simulink model "simulink_MPC2"  (R2022b)
settings: Solver=VariableStepAuto  StartTime=0.0  StopTime=Tsim  RelTol=1e-3
values from neighbouring files (symbols this model uses):
  A = [-a_til(2:end)' [eye(length(a_til)-2); zeros(1,length(a_til)-2)]]    [MPC_deadtime.m]    (also in MPC_diofant.m = [1 -0.8]; SS_MPC_irrestrito.m = A'; SS_MPC_restrito.m = A')
  B = [b(2:end)']    [MPC_deadtime.m]    (also in MPC_diofant.m = [0.4 0.6]; SS_MPC_irrestrito.m = B'; SS_MPC_restrito.m = B')
  D = [c(2:end)'-a_til(2:end)']    [MPC_deadtime.m]    (also in SS_MPC_irrestrito.m = D'; SS_MPC_restrito.m = D')
  DistAmplitude = -0.1    [MPC_SS.m]    (also in MPC_ex1_c1.m = 1; MPC_ex1_c2.m = 1; MPC_ex1_c3.m; MPC_ex2_c1.m = -1)
  F = zeros(N,length(a_)-1)    [MPC_SS.m]    (also in MPC_diofant.m = [F; r(2:end)]; MPC_ex1_c1.m; MPC_ex1_c2.m; MPC_ex1_c3.m)
  H = [1 zeros(1,Max-1)]    [MPC_deadtime.m]    (also in SS_MPC_irrestrito.m = H'; SS_MPC_restrito.m = H')
  K = K(1,:)    [MPC_SS.m]    (also in MPC_deadtime.m; MPC_diofant.m = aux(1,:); MPC_ex1_c1.m; MPC_ex1_c2.m)
  Kr = sum(K)    [MPC_SS.m]    (also in MPC_deadtime.m; MPC_diofant.m; MPC_ex1_c1.m; MPC_ex1_c2.m)
  RefAmplitude = 1    [MPC_SS.m]    (also in MPC_ex1_c1.m; MPC_ex1_c2.m; MPC_ex1_c3.m; MPC_ex2_c1.m)
  RefInitialValue = 0    [MPC_SS.m]    (also in MPC_ex1_c1.m; MPC_ex1_c2.m; MPC_ex1_c3.m; MPC_ex2_c1.m)
  Tdist = 20    [MPC_SS.m]    (also in MPC_deadtime.m = 15; MPC_ex1_c1.m; MPC_ex1_c2.m; MPC_ex1_c3.m)
  Tref = 0    [MPC_SS.m]    (also in MPC_ex1_c1.m; MPC_ex1_c2.m; MPC_ex1_c3.m; MPC_ex2_c1.m)
  Ts = 1    [MPC_SS.m]    (also in MPC_deadtime.m = 0.1; MPC_ex1_c1.m; MPC_ex1_c2.m; MPC_ex1_c3.m)
libraries: cstblocks x2
settings Model: Creator=gabrielfreitas  LastModifiedBy=sergio
settings SolverCC: AlgebraicLoopSolver=TrustRegion
settings DebuggingCC: UnconnectedInputMsg=warning  UnconnectedOutputMsg=warning  UnconnectedLineMsg=warning  SFMachineParentedDataDiag=warning
settings ModelReferenceCC: EnableRefExpFcnMdlSchedulingChecks=on

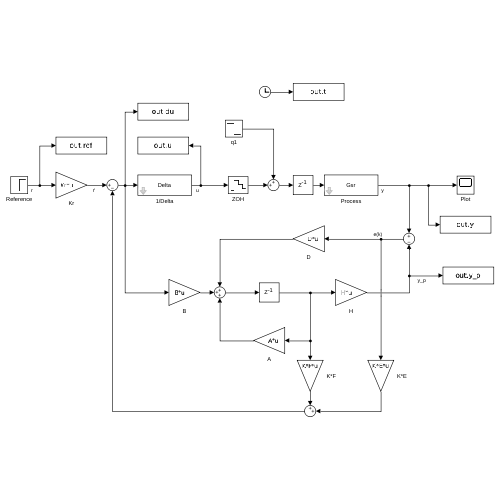
[thumbnail: Simulink's stored preview of the top-level diagram]
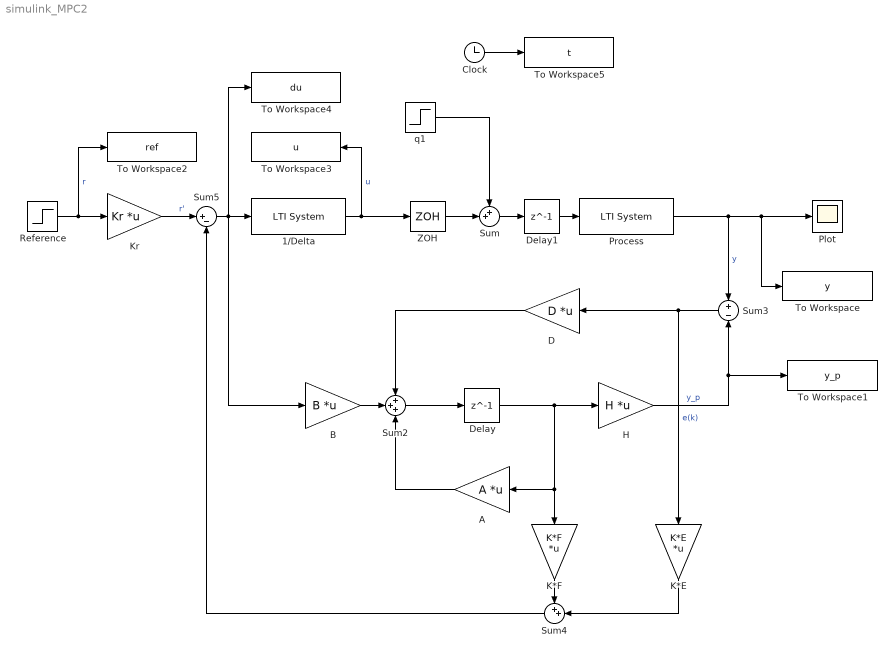
== system simulink_MPC2 ==
  1/Delta : cstblocks/LTI System  sys=Delta  IC=[]
  A : Gain  Gain=A  Multiplication=Matrix(K*u)
  B : Gain  Gain=B  Multiplication=Matrix(K*u)
  Clock : Clock
  D : Gain  Gain=D  Multiplication=Matrix(K*u)
  Delay : Delay  DelayLength=1  SampleTime=Ts
  Delay1 : Delay  DelayLength=1  SampleTime=Ts
  H : Gain  Gain=H  Multiplication=Matrix(K*u)
  K*E : Gain  Gain=K*E  Multiplication=Matrix(K*u)
  K*F : Gain  Gain=K*F  Multiplication=Matrix(K*u)
  Kr : Gain  Gain=Kr  Multiplication=Matrix(K*u)
  Plot : Scope
  Process : cstblocks/LTI System  sys=Gsr  IC=[]
  Reference : Step  Time=Tref  Before=RefInitialValue  After=RefAmplitude  SampleTime=0
  Sum : Sum  Inputs=++|
  Sum2 : Sum  Inputs=+++
  Sum3 : Sum  Inputs=+|-
  Sum4 : Sum  Inputs=++|
  Sum5 : Sum  Inputs=|+-
  To Workspace : ToWorkspace  VariableName=y  SampleTime=Ts
      settings: Save2DSignal=2-D array (concatenate along first dimension)
  To Workspace1 : ToWorkspace  VariableName=y_p  SampleTime=Ts
      settings: Save2DSignal=2-D array (concatenate along first dimension)
  To Workspace2 : ToWorkspace  VariableName=ref  SampleTime=Ts
      settings: Save2DSignal=2-D array (concatenate along first dimension)
  To Workspace3 : ToWorkspace  VariableName=u  SampleTime=Ts
      settings: Save2DSignal=2-D array (concatenate along first dimension)
  To Workspace4 : ToWorkspace  VariableName=du  SampleTime=Ts
      settings: Save2DSignal=2-D array (concatenate along first dimension)
  To Workspace5 : ToWorkspace  VariableName=t  SampleTime=Ts
      settings: Save2DSignal=2-D array (concatenate along first dimension)
  ZOH : ZeroOrderHold  SampleTime=Ts
  q1 : Step  Time=Tdist  After=DistAmplitude  SampleTime=0
  wires:
  q1/1 -> Sum/1
  ZOH/1 -> Sum/2
  1/Delta/1 -> To Workspace3/1, ZOH/1  "u"
  B/1 -> Sum2/2
  Sum3/1 -> D/1, K*E/1  "e(k)"
  D/1 -> Sum2/1
  Sum2/1 -> Delay/1
  Delay/1 -> A/1, K*F/1, H/1
  H/1 -> To Workspace1/1, Sum3/2  "y_p"
  A/1 -> Sum2/3
  K*E/1 -> Sum4/2
  K*F/1 -> Sum4/1
  Sum4/1 -> Sum5/2
  Kr/1 -> Sum5/1  "r'"
  Reference/1 -> To Workspace2/1, Kr/1  "r"
  Sum5/1 -> B/1, To Workspace4/1, 1/Delta/1
  Sum/1 -> Delay1/1
  Delay1/1 -> Process/1
  Clock/1 -> To Workspace5/1
  Process/1 -> Sum3/1, To Workspace/1, Plot/1  "y"
